simulink model "myModel_withoutRxTx"  (R2018b)
settings: Solver=FixedStepDiscrete  StartTime=0.0  StopTime=0.06  RelTol=1e-3  EnableMultiTasking=on
PreLoadFcn:
  | filepath = 'D:\Files\Ilya\Desktop\Аспирантура\Диссертация\Модель_канала\myModel'
  | addpath('D:\Files\Ilya\Desktop\Аспирантура\Диссертация\Модель_канала\myModel')
  | cd 'D:\Files\Ilya\Desktop\Аспирантура\Диссертация\Модель_канала\myModel'
  | load example_channel.mat
  | Fs = 6e5;
  | tmp = size(hmat);
  | hsamp = tmp(1);
  | timesamp = tmp(2);
  | upsamp = ceil(Fs/df/hsamp)*hsamp;
undefined symbols (not defined in the file): designMultirateFIR, dt, hmat
libraries: dspswit3 x3, dspindex x2, powerlib_meascontrol x1, dspmlti4 x1
settings Model: Creator=Ilya  LastModifiedBy=Ilya
settings SolverCC: AutoInsertRateTranBlk=on
settings OptimizationCC: BlockReduction=off  ConditionallyExecuteInputs=off  DefaultParameterBehavior=Inlined  UseDivisionForNetSlopeComputation=on  UseFloatMulNetSlope=on  UseSpecifiedMinMax=on  InlineInvariantSignals=on  PassReuseOutputArgsAs=Individual arguments  ZeroExternalMemoryAtStartup=off  ZeroInternalMemoryAtStartup=off  NoFixptDivByZeroProtection=on  EfficientFloat2IntCast=on  LifeSpan=1  OptimizeBlockOrder=speed  DifferentSizesBufferReuse=on
settings DebuggingCC: AlgebraicLoopMsg=error  ParameterTunabilityLossMsg=error
settings HardwareCC: ProdBitPerPointer=32  ProdBitPerSizeT=32  ProdBitPerPtrDiffT=32  ProdLargestAtomicFloat=None  ProdIntDivRoundTo=Undefined  ProdEndianess=Unspecified  ProdWordSize=32  ProdHWDeviceType=ASIC/FPGA->ASIC/FPGA  TargetBitPerPointer=64  TargetBitPerSizeT=64  TargetBitPerPtrDiffT=64  TargetLongLongMode=on  TargetIntDivRoundTo=Zero  TargetEndianess=LittleEndian  TargetWordSize=64  TargetHWDeviceType=Custom Processor->MATLAB Host Computer  ProdEqTarget=off
settings SFSimCC: MATLABDynamicMemAlloc=off
settings RTWCC: SystemTargetFile=ert.tlc  TemplateMakefile=ert_default_tmf  GenerateReport=on  BuildConfiguration=Faster Runs  IncludeHyperlinkInReport=on  LaunchReport=on  GenerateTraceInfo=on  GenerateTraceReport=on  GenerateTraceReportSl=on  GenerateTraceReportSf=on  GenerateTraceReportEml=on  GenerateCodeMetricsReport=on
settings CodeAppCC: ForceParamTrailComments=on  IgnoreCustomStorageClasses=off  OperatorAnnotations=on  SimulinkDataObjDesc=on  SFDataObjDesc=on  CustomSymbolStrGlobalVar=rt$N$M  CustomSymbolStrType=$N$M  CustomSymbolStrFcn=$N$M$F  CustomSymbolStrMacro=$N$M  InsertBlockDesc=on
settings ERTTargetCC: TargetLangStandard=C99 (ISO)  GenerateSampleERTMain=on  IncludeMdlTerminateFcn=off  CombineSignalStateStructs=on  SupportAbsoluteTime=off  SupportComplex=off  SupportNonInlinedSFcns=on  InlinedParameterPlacement=NonHierarchical  ERTCustomFileTemplate=example_file_process.tlc  ERTFilePackagingFormat=CompactWithDataFile

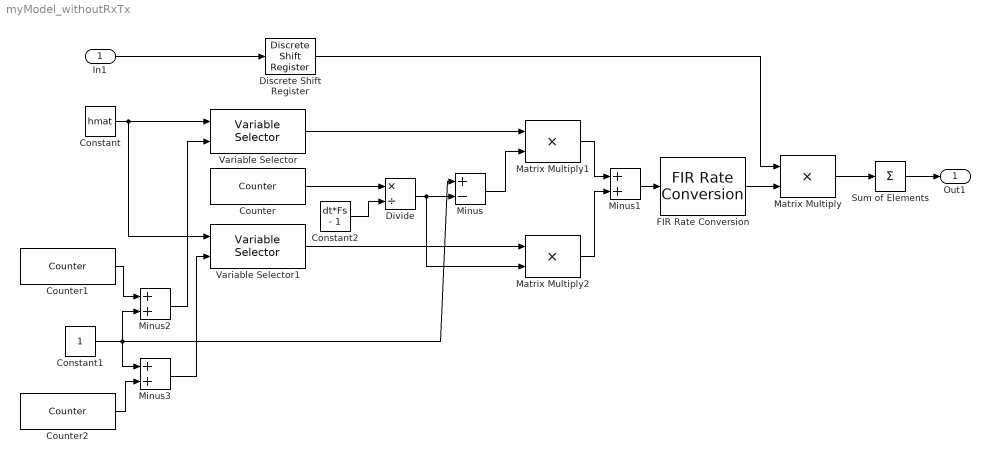
== system myModel_withoutRxTx ==
  In1 : Inport
  Constant : Constant  Value=hmat  VectorParams1D=off  SampleTime=-1
  Constant1 : Constant
  Constant2 : Constant  Value=dt*Fs - 1
  Counter : dspswit3/Counter  Direction=Up  CountEvent=Free running  CounterSize=User defined  MaxCount=dt*Fs - 1  InitialCount=0  Output=Count  HitValue=32  ResetInput=off  SamplesPerFrame=1  Ts=1/Fs  CntDtype=double  HitDtype=Logical
  Counter1 : dspswit3/Counter  Direction=Up  CountEvent=Free running  CounterSize=User defined  MaxCount=timesamp-1  InitialCount=0  Output=Count  HitValue=32  ResetInput=off  SamplesPerFrame=1  Ts=dt  CntDtype=double  HitDtype=Logical
  Counter2 : dspswit3/Counter  Direction=Up  CountEvent=Free running  CounterSize=User defined  MaxCount=timesamp-1  InitialCount=1  Output=Count  HitValue=32  ResetInput=off  SamplesPerFrame=1  Ts=dt  CntDtype=double  HitDtype=Logical
  Discrete Shift Register : powerlib_meascontrol/Additional Components/Discrete Shift Register  NSamples=upsamp  InitialValue=0  Ts=1/Fs
      settings: SourceProductName=Simscape Power Systems  SourceProductBaseCode=PS
  Divide : Product  Inputs=*/
  FIR Rate Conversion : dspmlti4/FIR Rate Conversion  FilterSource=Auto  L=upsamp  h=designMultirateFIR(3,2)  M=hsamp  FilterObject=FRC  roundingMode=Floor  overflowMode=off  firstCoeffDataTypeStr=Inherit: Same word length as input  firstCoeffMin=[]  firstCoeffMax=[]  firstCoeffLastDataTypeStr=Inherit: Same word length as input  outputDataTypeStr=Inherit: Same as accumulator  outputMin=[]  outputMax=[]  outputLastDataTypeStr=Inherit: Same as accumulator
      settings: SourceProductName=DSP System Toolbox  SourceProductBaseCode=DS
  Matrix Multiply : Product
  Matrix Multiply1 : Product
  Matrix Multiply2 : Product
  Minus : Sum  Inputs=+-
  Minus1 : Sum
  Minus2 : Sum
  Minus3 : Sum
  Sum of Elements : Sum  Inputs=+
  Variable Selector : dspindex/Variable Selector  NumInputs=1  rowsOrCols=Columns  IdxMode=Variable  Elements=[1 3]  ZerOneIdxMode=One-based  errmode=Clip Index  FillMode=on  FillValues=0
  Variable Selector1 : dspindex/Variable Selector  NumInputs=1  rowsOrCols=Columns  IdxMode=Variable  Elements=[1 3]  ZerOneIdxMode=One-based  errmode=Clip Index  FillMode=on  FillValues=0
  Out1 : Outport
  wires:
  Discrete Shift Register/1 -> Matrix Multiply/1
  Constant/1 -> Variable Selector1/1, Variable Selector/1
  Matrix Multiply/1 -> Sum of Elements/1
  FIR Rate Conversion/1 -> Matrix Multiply/2
  Variable Selector/1 -> Matrix Multiply1/1
  Variable Selector1/1 -> Matrix Multiply2/1
  Counter/1 -> Divide/1
  Constant2/1 -> Divide/2
  Divide/1 -> Matrix Multiply2/2, Minus/2
  Minus/1 -> Matrix Multiply1/2
  Matrix Multiply1/1 -> Minus1/1
  Matrix Multiply2/1 -> Minus1/2
  Minus1/1 -> FIR Rate Conversion/1
  Minus2/1 -> Variable Selector/2
  Counter1/1 -> Minus2/1
  Constant1/1 -> Minus3/1, Minus/1, Minus2/2
  Counter2/1 -> Minus3/2
  Minus3/1 -> Variable Selector1/2
  Sum of Elements/1 -> Out1/1
  In1/1 -> Discrete Shift Register/1
